simulink library "DAQ_lib_HallPositionTorque"  (R2014b)
settings: Solver=ode45  StartTime=0.0  StopTime=10.0  RelTol=1e-3
undefined symbols (not defined in the file): A_lpf_velocity, ANOMALY_INIT, B1_lpf_velocity, B2_lpf_velocity, Calibration, EnableFT, EncoderAngleLimits, EncoderFiltSys, EncoderThreshold, FTCalibration, GearOffsets, IMUAngleLimits, IMUCommand, IMUThreshold, IMUTorsoOffsets, m_XR17D15x, MAX_ANOMALY, MedullaCommand, MicrostrainFiltSys, MODBUS_TIMEOUT, ResetDAQ, ResetYaw, sample_time, standard, STREAMING_TIMEOUT, TareFT, TorsoCOMOffsets, Ts, TsCAN, TsKVH, UseMicrostrainRate
libraries: xpcethercatlib x207, simulink x53, canmsglib x21, speedgoatlib x13, slrtlib x5, speedgoatlib_IO601 x5, dspswit3 x2, dspmtrx3 x2, xpcseriallib x1, SpeedgoatModified x1
(part 7 of 7)

== stateflow chart DAQ_lib_HallPositionTorque/DAQ Safety Stops IMU Elmo Amplifiers Position and Torque Control with Hall Sensors/DAQ/SerialInterfaces/FTInterface/Subsystem/FTStateMachine ==
  state Run
    state FTSetup [parallel]
      settings: executionOrder=1
      state ModbusMode
        entry:
        clearModbusCommand();
        clearCalibration();
        RequestStreamingMode = 0;
        state SetSessionId
          entry:
          FTSetupStatus = 2;
        state ReadCalibration
          entry:
          clearCalibration();
          state SendRequest
            entry:
            FTSetupStatus = 3;
            requestCalibration();
            during:
            clearModbusCommand();
          state ParseRequest
            entry:
            FTSetupStatus = 4;
            parseCalibration();
          (default) -> SendRequest
          SendRequest -> ParseRequest [order 1] : [validResponse()]
          ParseRequest -> SendRequest [order 1] : [CalibrationBufferEnd<338]
          SendRequest -> SendRequest [order 2] : [after(0.2,sec)]
        state WriteActiveCalibration
          entry:
          FTSetupStatus = 1.30;
          (history)
          state LockStorage
            entry:
            FTSetupStatus = 8;
            lockUnlockStorage(0);
            during:
            clearModbusCommand();
          state writeActiveCal
            entry:
            FTSetupStatus = 7;
            writeActiveCalibration();
            during:
            clearModbusCommand();
          state readActiveCal
            entry:
            FTSetupStatus = 5;
            readActiveCalibration();
            during:
            clearModbusCommand();
          state UnlockStorage
            entry:
            FTSetupStatus = 6;
            lockUnlockStorage(1);
            during:
            clearModbusCommand();
          (default) -> readActiveCal
          writeActiveCal -> LockStorage : [validResponse()]
          LockStorage -> readActiveCal : [validResponse()]
          UnlockStorage -> writeActiveCal : [validResponse()]
          readActiveCal -> UnlockStorage [order 2] : [validResponse()]
        (default) -> SetSessionId
        SetSessionId -> ReadCalibration
        ParseRequest -> WriteActiveCalibration [order 2]
        WriteActiveCalibration -> WriteActiveCalibration : [after(2*MODBUS_TIMEOUT, sec)]
      state Initialize
        entry:
        FTSetupStatus = 0;
        clearModbusCommand();
        clearCalibration();
        RequestStreamingMode = 0;
      state StreamingMode
        entry:
        FTSetupStatus = 9;
        clearModbusCommand();
        RequestStreamingMode = 1;
      (default) -> Initialize
      Initialize -> Run.FTSetup.ModbusMode : [FTInterfaceStatus == 5]
      readActiveCal -> Run.FTSetup.StreamingMode [order 1] : [validResponse() && verifyActiveCalibration()]
    state FTInterface [parallel]
      settings: executionOrder=2
      state ModbusMode
        entry:
        clearGauge();
        clearSerialOut();
        state ModbusIdle
          entry:
          FTInterfaceStatus = 5;
          clearModbusResponse();
          clearSerialBuffer();
        state ModbusSend
          entry:
          FTInterfaceStatus = 6;
          clearSerialBuffer();
          sendModbusCmd(ModbusCommand);
          exit:
          clearSerialOut();
        state ModbusReceive
          entry, during:
          FTInterfaceStatus = 7;
          readModbusResponse()
        state ModbusValidate
          entry:
          FTInterfaceStatus = 8;
          validateModbusResponse();
          exit:
          clearModbusResponse();
        (default) -> ModbusIdle
        (junction 37) -> ModbusIdle
        (junction 99) -> (junction 37) [order 2]
        ModbusIdle -> ModbusSend [order 2] : [ModbusCommand(1)>0]
        (junction 99) -> ModbusSend [order 1] : [ModbusCommand(1)>0]
        (junction 36) -> (junction 99)
        ModbusSend -> ModbusReceive
        ModbusReceive -> (junction 36) [order 2] : [after(MODBUS_TIMEOUT, sec)]
        (junction 86) -> (junction 36)
        ModbusReceive -> ModbusValidate [order 1] : [Valid]
        ModbusValidate -> (junction 86)
      state InitializeStreaming
        entry:
        FTInterfaceStatus = 3;
        clearSerialBuffer();
        sendStreamingCmd(1);
        exit:
        clearSerialOut();
      state CheckStreaming
        state WaitClear
          entry:
          FTInterfaceStatus = 1;
          clearSerialOut();
          clearSerialBuffer();
        state CheckSerialInput
          entry:
          FTInterfaceStatus = 2;
        (default) -> WaitClear
        WaitClear -> CheckSerialInput
      state StreamingMode
        entry:
        FTInterfaceStatus = 9;
        clearGauge();
        clearSerialOut();
        clearSerialBuffer();
        during:
        parseStreamingData();
      state EndStreaming
        entry:
        FTInterfaceStatus = 4;
        clearSerialBuffer();
        sendStreamingCmd(0);
        exit:
        clearSerialOut();
      ModbusIdle -> InitializeStreaming [order 1] : [RequestStreamingMode ~= 0]
      InitializeStreaming -> CheckStreaming
      (default) -> CheckStreaming
      CheckSerialInput -> Run.FTInterface.ModbusMode [order 2] : [after(STREAMING_TIMEOUT, sec)]
      CheckSerialInput -> Run.FTInterface.StreamingMode [order 1] : [SerialIn(1)>0]
      EndStreaming -> CheckStreaming
      Run.FTInterface.StreamingMode -> EndStreaming : [RequestStreamingMode==0]
  state Reset
    entry:
    FTSetupStatus = 0;
    FTInterfaceStatus = 0;
    clearModbusCommand();
    clearModbusResponse();
    clearCalibration();
    clearGauge();
    clearSerialBuffer();
    clearSerialOut();
  (default) -> Reset
  Reset -> Run : [Reset==0]
  Run -> Reset : [Reset>0]
  data: valid function_output; Unlock function_input; ok function_output; Command function_input; Select function_input; CalibrationSet input; Reset input; RequestStreamingMode local; SerialBuffer local; SerialBufferEnd local; GaugeStatus output; Gauge output; Calibration output Bus: FTCalibrationBus; ModbusCommand local; ModbusResponse local; FTInterfaceStatus output; SerialIn input; ResponseLength local; LastModbusFunction local; MODBUS_TIMEOUT parameter; STREAMING_TIMEOUT parameter; Valid local; FTSetupStatus output; SerialOut output; FTCalibration parameter Bus: FTCalibrationBus; CalibrationBuffer local; CalibrationBufferEnd local
  function requestCalibration:
    | function requestCalibration() %#codegen
    |    % ATI F/T Calibration data are stored in 16-bit holding registers. There
    |    % are 16 calibration sets, each 338 bytes (or 169 registers) long. They
    |    % are stored beginning at holding register address 0x00e3 (Calibration
    |    % 1). Subsequent calibration sets are spaced 192 holding registers
    |    % apart.
    |    BaseAddress = uint32(hex2dec('00e3')) + uint32(192 * (CalibrationSet - 1));
    |    
    |    % Calibration data must be read in two or more parts due to length
    |    % restricitons in the Modbus protocol. In order to keep buffer sizes
    |    % small we'll read in parts of no more than 12 registers each.
    |    
    |    NextCalibrationRegister = uint32(CalibrationBufferEnd/2);
    |    Address = BaseAddress + NextCalibrationRegister;
    |    NumRegs = min(12, 169 - NextCalibrationRegister);
    |    
    |    ModbusFunction = 3;
    |    ModbusCommand(1:6) = uint32([5; ModbusFunction; bitshift(Address,-8); bitand(Address,255); 0; NumRegs]);
    | end
  function parseCalibration:
    | function parseCalibration() %#codegen
    |     % Calibration data must be read in two or more parts due to length
    |     % restricitons in the Modbus protocol.
    |     
    |     NumBytes = min(ModbusResponse(3), length(CalibrationBuffer) - CalibrationBufferEnd);
    |     CalibrationBuffer(CalibrationBufferEnd+(1:NumBytes)) = ModbusResponse(3+(1:NumBytes));
    |     CalibrationBufferEnd = CalibrationBufferEnd + NumBytes;
    |     if (CalibrationBufferEnd==338)
    |         Calibration = parseFTCalibration2(CalibrationBuffer(1:CalibrationBufferEnd));
    |     end
    | end
    | 
    | function Cal = parseFTCalibration2(CalibrationBuffer)
    |     Cal.CalibSerialNumber = parseUint8(CalibrationBuffer(1:8));
    |     Cal.CalibPartNumber   = parseUint8(CalibrationBuffer(9:40));
    |     Cal.CalibFamilyId     = parseUint8(CalibrationBuffer(41:44));
    |     Cal.CalibTime         = parseUint8(CalibrationBuffer(45:64));
    |     Cal.BasicMatrix       = reshape(parseFloat(CalibrationBuffer(65:208)), 6, 6).';
    |     Cal.ForceUnits        = parseUint8(CalibrationBuffer(209));
    |     Cal.TorqueUnits       = parseUint8(CalibrationBuffer(210));
    |     Cal.MaxRating         = parseFloat(CalibrationBuffer(211:234));
    |     Cal.CountsPerForce    = parseInt32(CalibrationBuffer(235:238));
    |     Cal.CountsPerTorque   = parseInt32(CalibrationBuffer(239:242));
    |     Cal.GageGain          = parseUint16(CalibrationBuffer(243:254));
    |     Cal.GageOffset        = parseUint16(CalibrationBuffer(255:266));
    |     Cal.Resolution        = parseUint8(CalibrationBuffer(267:272));
    |     Cal.Range             = parseUint8(CalibrationBuffer(273:278));
    |     Cal.ScaleFactor16     = parseUint16(CalibrationBuffer(279:290));
    |     Cal.UserField1        = parseUint8(CalibrationBuffer(291:306));
    |     Cal.UserField2        = parseUint8(CalibrationBuffer(307:322));
    |     Cal.SpareData         = parseUint8(CalibrationBuffer(323:338));
    | end
    | 
    | 
    | function d = parseUint8(D)
    |     d = double(D);
    | end
    | 
    | function d = parseFloat(D)
    |     D1 = uint32(D);
    |     D2 = bitshift(D1(1:4:end), 24) + bitshift(D1(2:4:end), 16) + bitshift(D1(3:4:end), 8) + D1(4:4:end);
    |     d = double(typecast(D2, 'single'));
    | end
    | 
    | function d = parseUint32(D)
    |     D1 = uint32(D);
    |     D2 = bitshift(D1(1:4:end), 24) + bitshift(D1(2:4:end), 16) + bitshift(D1(3:4:end), 8) + D1(4:4:end);
    |     d  = double(D2);
    | end
    | 
    | function d = parseInt32(D)
    |     D1 = int32(D);
    |     D2 = bitshift(D1(1:4:end), 24) + bitshift(D1(2:4:end), 16) + bitshift(D1(3:4:end), 8) + D1(4:4:end);
    |     d  = double(D2);
    | end
    | 
    | function d = parseUint16(D)
    |     D1 = uint16(D);
    |     D2 = bitshift(D1(1:2:end), 8) + D1(2:2:end);
    |     d  = double(D2);
    | end
  function valid = validResponse:
    | function valid = validResponse %#codegen
    |     valid = false;
    |     
    |     ModbusFunction = double(ModbusResponse(2));
    |     
    |     if (ModbusResponse(1) > 1)    
    |         switch ModbusFunction
    |             case {3, 6, 16}
    |                 % 3: Read holding registers
    |                 % 6: Write single register
    |                 % 16: Write multiple registers
    |                 
    |                 % If there were an error, the response ModbusFunction code
    |                 % would be (F + 0x80
    |                 valid = true;
    |                 
    |             case {70, 106}
    |                 ModbusByteCount = double(ModbusResponse(3));
    |                 valid = (ModbusByteCount == 1);
    |         end
    |     end
    | end
  function lockUnlockStorage(Unlock):
    | function lockUnlockStorage(Unlock) %#codegen
    |     % ATI F/T Calibration data are stored in holding registers. After
    |     % reading a calibration data set, we must write the GaugeGain and
    |     % GaugeOffset values to the active gain and offset holding registers.
    |     % Before writing to the active gain/offset registers, we must unlock
    |     % the storage.
    |     
    |     ModbusFunction = 106; % Read holding registers
    |     if (Unlock==1)
    |         Data = 170; % hex2dec('aa')
    |     else
    |         Data = 24; % hex2dec('18')
    |     end
    |         
    |     ModbusCommand(1:3) = uint32([2; ModbusFunction; Data]);
    | end
  function readActiveCalibration:
    | function readActiveCalibration %#codegen
    |     % ATI F/T Calibration data are stored in holding registers. After
    |     % reading a calibration data set, we must write the GaugeGain and
    |     % GaugeOffset values to the active gain and offset holding registers.
    |     % Holding register addresses:
    |     %   0x0000-0x0005 Active Gain pots
    |     %   0x0006-0x000B Active Offset DACs
    |     ModbusFunction = 3; % Read holding registers
    |     Address = uint32(0);
    |     NumRegs = 12;
    |     ModbusCommand(1:6) = uint32([5; ModbusFunction; bitshift(Address,-8); bitand(Address,255); 0; NumRegs]);
    | end
  function ok = verifyActiveCalibration:
    | function ok = verifyActiveCalibration %#codegen
    |     % ATI F/T Calibration data are stored in holding registers. After
    |     % reading a calibration data set, we must write the GaugeGain and
    |     % GaugeOffset values to the active gain and offset holding registers.
    |     % Holding register addresses:
    |     %   0x0000-0x0005 Active Gain pots
    |     %   0x0006-0x000B Active Offset DACs
    |     ok = false;
    |     
    |     % Check response length
    |     ActualResponseLength = double(ModbusResponse(1));
    |     if (ActualResponseLength ~= 26)
    |         return
    |     end
    |     
    |     % Compare gain and offset values with those in the calibration
    |     % structure
    |     ActiveGaugeGain   = parseUint16(ModbusResponse(3  + (1:12)));
    |     ActiveGaugeOffset = parseUint16(ModbusResponse(15 + (1:12)));
    |     
    |     if any(ActiveGaugeGain ~= Calibration.GageGain) ...
    |             || any(ActiveGaugeOffset ~= Calibration.GageOffset)
    |         return;
    |     end
    |     
    |     % Then it looks okay
    |     ok = true;
    | end
    | 
    | function u = parseUint16(D)
    |     D1 = double(D);
    |     u = D1(1:2:end)*256 + D1(2:2:end);
    | end
  function writeActiveCalibration:
    | function writeActiveCalibration %#codegen
    |     % ATI F/T Calibration data are stored in holding registers. After
    |     % reading a calibration data set, we must write the GaugeGain and
    |     % GaugeOffset values to the active gain and offset holding registers.
    |     % Holding register addresses:
    |     %   0x0000-0x0005 Active Gain pots
    |     %   0x0006-0x000B Active Offset DACs
    |     ModbusFunction = 16; % Write multiple registers
    |     Address = uint32(0);
    |     NumRegs = 12;
    |     
    |     ModbusCommand(1:31) = uint32([30; ModbusFunction; bitshift(Address,-8); bitand(Address,255); 0; NumRegs; 2*NumRegs; zeros(2*NumRegs, 1, 'uint32')]);
    |     
    |     Data = uint32([Calibration.GageGain Calibration.GageOffset]);
    |     for k=1:NumRegs
    |         ModbusCommand(8 + 2*(k-1)) = bitshift(Data(k), -8); 
    |         ModbusCommand(9 + 2*(k-1)) = bitand(Data(k), 255);
    |     end
    | end
  function parseStreamingData:
    | function parseStreamingData %#codegen
    |     % Look for the last good F/T packet in the SerialIn buffer.
    |     % See section 9.4.2 of 9620-05-Digital FT______________Last_version_300414.pdf at
    |     % https://sites.google.com/a/umich.edu/atrias/knowledge-base/hardware/load-cells
    |     %
    |     % GaugeStatus is a scalar:
    |     %   GaugeStatus = -1   if no valid packets found (no valid checksum)
    |     %   GaugeStatus = 1    if a valid packet was found but the gauge status
    |     %                      bit was set (indicates a strain gauge error)
    |     %   GaugeStatus = 0    if a good packet was found
    |     
    |     Gauge = zeros(6,1);
    |     GaugeStatus = -1;
    |     
    |     numNewBytes = min(SerialIn(1), length(SerialIn)-1);
    |     k = 1;
    |     while (k + 13 <= numNewBytes)
    |         % Verify checksum (first seven bits of last byte in packet)
    |         valid = CheckSample(SerialIn(k+(1:13)));
    |         
    |         if valid
    |             % Get gauge status bit (msb of last byte in packet) if the packet is valid
    |             StatusBit = double(bitget(SerialIn(k+13), 8));
    |             if (StatusBit == 0) || (GaugeStatus == -1)
    |                 Gauge     = ComputeGauge(SerialIn(k+(1:12)));
    |                 GaugeStatus = StatusBit;
    |             end
    |             k = k + 13;
    |         else
    |             k = k + 1;
    |         end 
    |     end
    | end
    | 
    | function valid = CheckSample( sampleBytes )
    |     checkSum = sum(int16(sampleBytes(1:12)), 'native');
    |     valid = bitand(checkSum, 127) == bitand(sampleBytes(13), 127);
    | end
    | 
    | function Gauge = ComputeGauge(D)
    |     % Convert uint8 to int16 and reorder
    |     % The Digital F/T board returns Gauge data in the order
    |     %   [G0 G2 G4 G1 G3 G5]'.
    |     % and we want it in the order
    |     %   [G0 G1 G2 G3 G4 G5].'
    |     
    |     Gauge = double( bitshift(int16(D([1 3 5 7 9 11])), 8) + int16(D([2 4 6 8 10 12])) );
    |     Gauge = Gauge([1 4 2 5 3 6]);
    | end
  function sendModbusCmd(Command):
    | function sendModbusCmd(Command) %#codegen
    |     
    |     % All ATI Digital F/T interface boards use Modbus address 10.
    |     % See ATI Digital F/T System Installation and Operation Manual
    |     % (Document #9620-05-Digital FT).
    |     L = Command(1);
    |     assert(L < 65);
    |     
    |     ModbusAddress  = uint32(10);
    |     ModbusFunction = Command(2);
    |     ModbusData     = Command(1+(2:L));
    |     ModbusPacket   = createModbusPacket32(ModbusAddress, ModbusFunction, ModbusData);
    |     
    |     L = length(ModbusPacket);
    |     SerialOut(1)     = uint32(L);
    |     SerialOut(2:L+1) = ModbusPacket;
    |     
    |     % Expected response length
    |     ResponseLength = getModbusResponseLength32(ModbusFunction, ModbusData);
    |     
    |     % Capture function
    |     LastModbusFunction = ModbusFunction;
    | end
  function readModbusResponse:
    | function readModbusResponse %#codegen
    |     % Insert the new data into the SerialBuffer
    |     numNewBytes = min(SerialIn(1), 256);
    |     assert(numNewBytes < 257);
    |     SerialBuffer(SerialBufferEnd + (1:numNewBytes)) = SerialIn(1 + (1:numNewBytes));
    |     SerialBufferEnd = SerialBufferEnd + numNewBytes;
    |     
    |     Valid = false; % Invalid packet
    |     if (SerialBuffer(2) == LastModbusFunction) && (SerialBufferEnd == 3 + ResponseLength)
    |         Valid = true; % Okay
    |     elseif (SerialBuffer(2) == LastModbusFunction+128) && (SerialBufferEnd == 5)
    |         Valid = true; % Exception
    |     end
    | 
    | end
  function sendStreamingCmd(Select):
    | function sendStreamingCmd(Select) %#codegen
    |     
    |     Function = uint16(70);
    |     if (Select==1)
    |         L = 2;
    |         Data = 85;
    |     else
    |         L = 16;
    |         Data = 85*ones(L-1,1,'uint32'); % JAMMING SEQUENCE
    |     end
    |     sendModbusCmd(uint32([L; Function; Data])) %#codegen
    | end
  function validateModbusResponse:
    | function validateModbusResponse %#codegen
    |     Valid = false;
    |     ModbusResponse = zeros(256, 1, 'uint32');
    |     
    |     if (SerialBuffer(2) == LastModbusFunction) && (SerialBufferEnd == 3 + ResponseLength) ...
    |             || (SerialBuffer(2) == LastModbusFunction + 128) && (SerialBufferEnd == 5)
    |         
    |         Valid = checkModbusCRC32(SerialBuffer(1:SerialBufferEnd));
    |         if Valid
    |             % Strip off the Modbus Address and CRC
    |             L = SerialBufferEnd-3;
    |             assert(L < 255);
    |             ModbusResponse(1) = uint32(L);
    |             ModbusResponse(1+(1:L)) = SerialBuffer(1+(1:L));
    |         end
    |     end
    | end
  function clearModbusCommand:
    | function clearModbusCommand %#codegen
    |     ModbusCommand = zeros(65, 1, 'uint32');
    | end
  function clearCalibration:
    | function clearCalibration %#codegen
    |     Calibration       = FTCalibration;
    |     CalibrationBuffer = zeros(512, 1, 'uint32');
    |     CalibrationBufferEnd = uint32(0);
    | end
  function clearSerialOut:
    | function clearSerialOut %#codegen
    |     SerialOut = zeros(65, 1, 'uint32');
    | end
  function clearModbusResponse:
    | function clearModbusResponse %#codegen
    |     ModbusResponse(1) = uint32(0);
    |     ModbusStatus = 0;
    | end
  function clearSerialBuffer:
    | function clearSerialBuffer %#codegen
    |     SerialBuffer = zeros(512, 1, 'uint32');
    |     SerialBufferEnd = uint32(0);
    | end
  function clearGauge:
    | function clearGauge %#codegen
    |     Gauge = zeros(6,1);
    |     GaugeStatus = 0;
    | end

== matlab function DAQ_lib_HallPositionTorque/DAQ Safety Stops IMU Elmo Amplifiers Position and Torque Control with Hall Sensors/DAQ/SerialInterfaces/KVH/ComputeEulerAngles ==
  data: RkIn input; wk input; RCal input; Reset input; R0In input; ZYX output; dZYX output; Rk output; R0 output; YawRolloverIn input; YawRollover output
function [ZYX, dZYX, Rk, R0, YawRollover] = fcn(RkIn, wk, RCal, Reset, R0In, YawRolloverIn) %#codegen
    % Convert from IMU frame to robot frame and compute Euler angles. The
    % yaw angle is zeroed whenever (Reset) is true.
        
    if (Reset)
        % Compute the rotation matrix which zeroes the initial yaw
        qT0 = M_to_ZYX(RkIn*RCal);
        R0  = Rz(-qT0(1));
    else
        R0 = R0In;
    end
    
    % Transform from IMU to robot frame and zero initial yaw
    Rk = R0*RkIn*RCal;
    
    % Convert Rk to ZYX Euler angles
    ZYX = M_to_ZYX(Rk);
    
    % Unroll yaw
    YawRolloverCount = YawRolloverIn(1);
    PreviousYaw      = YawRolloverIn(2);
    CurrentYaw       = ZYX(1);
    YawRolloverCount = YawRolloverCount + getYawRollover(CurrentYaw, PreviousYaw);
    YawRollover      = [YawRolloverCount; CurrentYaw];
    ZYX(1)           = ZYX(1) + 2*pi*YawRolloverCount;
    
    % Compute Euler angle derivatives
    qzT = ZYX(1);
    qyT = ZYX(2);
    
    if cos(qyT)>1e-3
        dZYX = [0 -sin(qzT) cos(qzT)*cos(qyT); 0 cos(qzT) sin(qzT)*cos(qyT); 1 0 -sin(qyT)]\(R0*RkIn*wk);
    else
        dZYX = [0; 0; 0];
    end
end

function R = Rz(t)
    R = [cos(t) -sin(t) 0; sin(t) cos(t) 0; 0 0 1];
end

function Rollover = getYawRollover(CurrentYaw, PreviousYaw)
    % Determine if a rollover has occurred on yaw angle If a rollover is
    % detected, the output Rollover is either +1 or -1, depending on the
    % direction of the rollover.
  
    if (PreviousYaw>0 && CurrentYaw < (PreviousYaw-pi))
        Rollover = 1;
    elseif (PreviousYaw<0 && CurrentYaw > (PreviousYaw+pi))
        Rollover = -1;
    else
        Rollover = 0;
    end
end

== matlab function DAQ_lib_HallPositionTorque/DAQ Safety Stops IMU Elmo Amplifiers Position and Torque Control with Hall Sensors/DAQ/SerialInterfaces/KVH/UpdateOrientation/EstimateOrientation ==
  data: DeltaAngle input; Acceleration input; Status input; Sequence input; Reset input; Rk output; wk output; Rkm1 input; wkm1 input; Akm1 input; Ak output; Seqkm1 input; Seqk output
function [Rk, wk, Ak, Seqk] = fcn(DeltaAngle,Acceleration,Status,Sequence,Reset,Rkm1,wkm1,Akm1,Seqkm1) %#codegen
    [Rk, wk, Ak, Seqk] = estimateOrientation(DeltaAngle,Acceleration,Rkm1,wkm1,Akm1,Status,Sequence,Seqkm1,Reset);
end

== matlab function DAQ_lib_HallPositionTorque/DAQ Safety Stops IMU Elmo Amplifiers Position and Torque Control with Hall Sensors/DAQ/SerialInterfaces/KVH/UpdateOrientation/MATLAB Function ==
  data: P input; Rotation output; Acceleration output; Status output; Sequence output; Temperature output; Valid output
function [Rotation,Acceleration,Status,Sequence,Temperature,Valid] = KVHParsePacket(P)
    %#codegen
    CMD = [254; 129; 255; 85]; %hex2dec(['FE';'81';'FF';'55']);
    
    Valid = false;
    if all(P(1:4) == CMD)
        Valid = kvhCheckCRC(P(1:36));
    end
    
    Rotation = parseSingle(P(5:16,:));
    Acceleration = parseSingle(P(17:28,:));
    Status = P(29);
    Sequence = double(P(30));
    Temperature = parseInt16(P(31:32));
end

function S = parseSingle(D)
    Stmp1 = uint32(reshape(D,4,[]));
    Stmp2 = 16777216*Stmp1(1,:) + 65536*Stmp1(2,:) + 256*Stmp1(3,:) + Stmp1(4,:);
    Stmp3 = typecast(Stmp2,'single');
    S = double(Stmp3');
end

function S = parseInt16(D)
    Stmp1 = uint16(reshape(D,2,[]));
    Stmp2 = 256*Stmp1(1,:) + Stmp1(2,:);
    S = double(Stmp2');
end

== matlab function DAQ_lib_HallPositionTorque/DAQ Safety Stops IMU Elmo Amplifiers Position and Torque Control with Hall Sensors/DAQ/StateEstimator/GeneralizedCoordinates ==
  data: EncoderAngles input; EncoderVelocities input; q_clean output; IMUAngles input; IMUVelocities input; UseMotorIncEncoders input; UseIMU input; dq_clean output; IMUTorsoOffset input; GearOffset input; Reset input
function [q_clean, dq_clean] = coords(EncoderAngles, EncoderVelocities, IMUAngles, IMUVelocities, UseMotorIncEncoders, UseIMU, IMUTorsoOffset, GearOffset, Reset)
    %#codegen
    
    % q_clean =
    %  [qzT; qyT; qxT; q1R; q2R; q1L; q2L; qgr1R; qgr2R; q3R; qgr1L; qgr2L; q3L];
    %
    % EncoderAngles = 
    %  [Leg1R; Leg2R; Leg1L; Leg2L; Motor1R; Motor2R; Motor1L; Motor2L; Hip3R; Hip3L; ...   % ABSOLUTE ENCODERS
    %   Inc1R; Inc2R; Inc1L; Inc2L; Inc3R; Inc3L; Boom; Boom; Boom]                         % INCREMENTAL ENCODERS
    
    if (Reset)
        q_clean  = zeros(13,1);
        dq_clean = zeros(13,1);
    else 
        q_clean  = EncoderAngles([17:19 1:6 15 7:8 16]);
        dq_clean = EncoderVelocities([17:19 1:6 15 7:8 16]);
        
        if (UseMotorIncEncoders)
            if 0
                q_clean([8:9 11:12])  = EncoderAngles(11:14)/50;
                dq_clean([8:9 11:12]) = EncoderVelocities(11:14)/50;
                
            elseif 0
                % BGB 2014-08-29
                % The incremental encoder on q1L was destroyed in the 60V
                % power fault event, so it cannot be used until it is
                % replaced.
                q_clean([8:9 12])  = EncoderAngles([11:12 14])/50;
                dq_clean([8:9 12]) = EncoderVelocities([11:12 14])/50;

            else
                % BGB 2015-02-05
                % Perhaps the harmonic drive is bad? We are seeing drift in
                % the 2L incremental motor encoder.
                q_clean(8:9)  = EncoderAngles(11:12)/50;
                dq_clean(8:9) = EncoderVelocities(11:12)/50;
            end
        end
        
        % Add offset to gear angles to allow zeroing of spring deflections.
        q_clean([8:9 11:12]) = q_clean([8:9 11:12]) + GearOffset*pi/180;
        
        if (UseIMU)
            q_clean(1:3)  = IMUAngles + [0; IMUTorsoOffset]*pi/180;
            dq_clean(1:3) = IMUVelocities;
        end
    end
end

== matlab function DAQ_lib_HallPositionTorque/DAQ Safety Stops IMU Elmo Amplifiers Position and Torque Control with Hall Sensors/FindHallOffsets ==
  data: q_in input; offsets output; hallPosition input
function offsets = fcn(q_in, hallPosition)
    %#codegen
    % HallPosition: 1R,2R,1L,2L
    q = q_in(8:13);
    scale = (1/10)*pi/180;
    
    offsets = q - scale*hallPosition;
end

== matlab function DAQ_lib_HallPositionTorque/DAQ Safety Stops IMU Elmo Amplifiers Position and Torque Control with Hall Sensors/SAFETY ==
  data: MotorCurrentCommand input; MotorCurrentCommandSafe output; MedullaCommand input; RequestSoftStop input; q input; dq input; Switches input; Thermistors input; SafetyCountIn input; MedullaCommandSafe output; SafetyState output; SafetyCountOut output; FaultDetected input
function [MotorCurrentCommandSafe, MedullaCommandSafe, SafetyState, SafetyCountOut] = SafetyCheck(MotorCurrentCommand, MedullaCommand, RequestSoftStop, q, dq, Switches, Thermistors, SafetyCountIn, FaultDetected)
    IMUCommand = 1; % Legacy.
    LogicVoltage = []; % Not currently used.
    SelectBasicLimits = 2;
    [MotorCurrentCommandSafe, MedullaCommandSafe, IMUCommandSafe, SafetyState, SafetyCountOut] = MARLOSafety(MotorCurrentCommand, MedullaCommand, IMUCommand, q, dq, Switches, Thermistors, LogicVoltage, SafetyCountIn, RequestSoftStop, SelectBasicLimits, FaultDetected);
end
